simulink model "lab3_step7"  (R2019b)
settings: Solver=VariableStepAuto  StartTime=0.0  StopTime=stop_time  RelTol=1e-3
InitFcn:
  | sm_callback_init
StopFcn:
  | y_out = output_signal.Data(:);
  | plot(y_out)
  | soundsc(y_out,Fs)
values from neighbouring files (symbols this model uses):
  mp = sm_init_avalon_signals(mp)    [sm_callback_init.m]
settings Model: Creator=yassi  LastModifiedBy=yassi
settings DataIOCC: ReturnWorkspaceOutputs=off

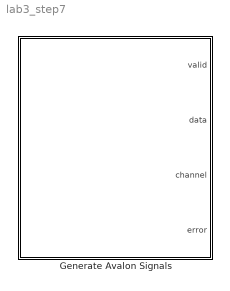
== system lab3_step7 ==
  Generate Avalon Signals : Subsystem

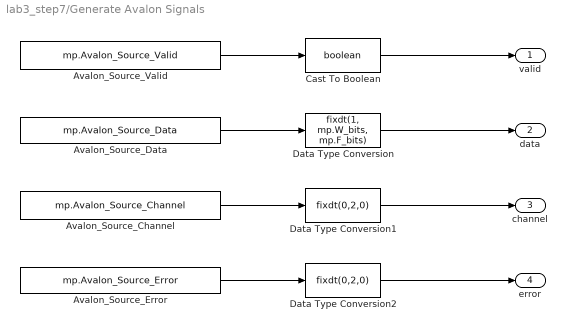
== system lab3_step7/Generate Avalon Signals ==
  Avalon_Source_Channel : FromWorkspace  VariableName=mp.Avalon_Source_Channel  OutDataTypeStr=double  SampleTime=mp.Ts_system
  Avalon_Source_Data : FromWorkspace  VariableName=mp.Avalon_Source_Data  OutDataTypeStr=double  SampleTime=mp.Ts_system
  Avalon_Source_Error : FromWorkspace  VariableName=mp.Avalon_Source_Error  OutDataTypeStr=double  SampleTime=mp.Ts_system
  Avalon_Source_Valid : FromWorkspace  VariableName=mp.Avalon_Source_Valid  OutDataTypeStr=double  SampleTime=mp.Ts_system
  Cast To Boolean : DataTypeConversion  OutDataTypeStr=boolean
  Data Type Conversion : DataTypeConversion  OutDataTypeStr=fixdt(1, mp.W_bits, mp.F_bits)
  Data Type Conversion1 : DataTypeConversion  OutDataTypeStr=fixdt(0,2,0)
  Data Type Conversion2 : DataTypeConversion  OutDataTypeStr=fixdt(0,2,0)
  valid : Outport
  data : Outport  Port=2
  channel : Outport  Port=3
  error : Outport  Port=4
  wires:
  Avalon_Source_Valid/1 -> Cast To Boolean/1
  Avalon_Source_Data/1 -> Data Type Conversion/1
  Avalon_Source_Channel/1 -> Data Type Conversion1/1
  Avalon_Source_Error/1 -> Data Type Conversion2/1
  Cast To Boolean/1 -> valid/1
  Data Type Conversion/1 -> data/1
  Data Type Conversion1/1 -> channel/1
  Data Type Conversion2/1 -> error/1
